simulink model "Test_thermal_rectifier_Werl"  (R2022a)
settings: Solver=VariableStepAuto  StartTime=0.0  StopTime=1000.0  RelTol=1e-3
libraries: nesl_utility x9
settings Model: Creator=Ravi  LastModifiedBy=Ravi

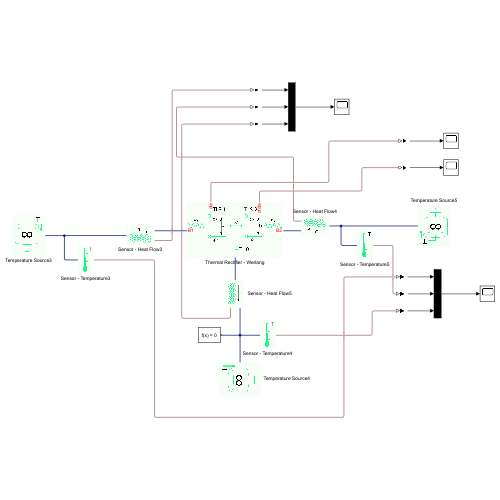
[thumbnail: Simulink's stored preview of the top-level diagram]
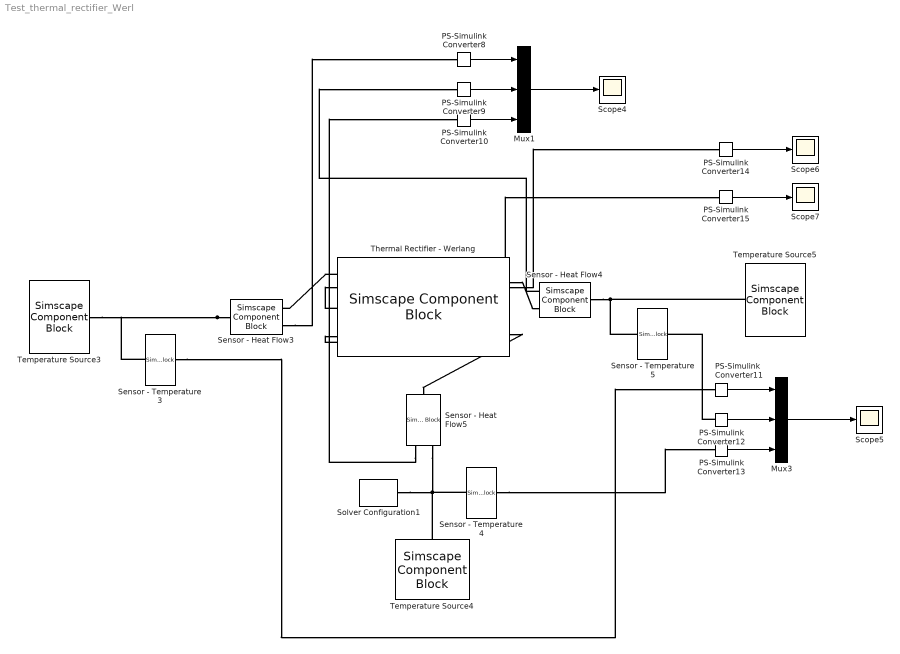
== system Test_thermal_rectifier_Werl ==
  Mux1 : Mux  Inputs=3
  Mux3 : Mux  Inputs=3
  PS-Simulink Converter{8..15} (8 alike) : nesl_utility/PS-Simulink Converter  PhysicalDomain=network_engine_domain  SubClassName=ps_output  LeftPortType=input  RightPortType=output  PseudoPeriodic=off  Frequencies=[]  VectorFormat=inherit  Unit=inherit  AffineConversion=off
      settings: SourceProductBaseCode=SS,PW,VE
  Scope{4..7} (4 alike) : Scope
  Sensor - Heat Flow3 : SimscapeComponentBlock  SourceFile=sensor_heat_flow  ComponentPath=sensor_heat_flow  ComponentVariants="[\"sensor_heat_flow\"]"  ComponentVariantNames="[\"sensor_heat_flow\"]"  ClassName=sensor_heat_flow  SchemaVersion=1  J_specify=off  J_priority=None  J=0  J_nominal_specify=off  J_nominal_unit=1  J_nominal_value=1
      settings: CopyFcn=simscape.engine.sli.internal.componentblockcallback(gcbh,'COPY')  PreCopyFcn=simscape.engine.sli.internal.componentblockcallback(gcbh,'PRECOPY')  PreDeleteFcn=simscape.engine.sli.internal.componentblockcallback(gcbh,'PREDELETE')  InternalSimscapePortConfiguration="{\"Bottom\":[],\"Left\":[{\"id\":\"inp\",\"label\":\"\",\"type\":\"quantum_thermal\"}],\"Right\":[{\"id\":\"out\",\"label\":\"\",\"type\":\"quantum_thermal\"},{\"id\":\"sense\",\"label\":\"\",\"type\":\"output\"}],\"Top\":[]}"
      mask Type: Heat flow rate sensor
  Sensor - Heat Flow4 : SimscapeComponentBlock  SourceFile=sensor_heat_flow  ComponentPath=sensor_heat_flow  ComponentVariants="[\"sensor_heat_flow\"]"  ComponentVariantNames="[\"sensor_heat_flow\"]"  ClassName=sensor_heat_flow  SchemaVersion=1  J_specify=off  J_priority=None  J=0  J_nominal_specify=off  J_nominal_unit=1  J_nominal_value=1
      settings: CopyFcn=simscape.engine.sli.internal.componentblockcallback(gcbh,'COPY')  PreCopyFcn=simscape.engine.sli.internal.componentblockcallback(gcbh,'PRECOPY')  PreDeleteFcn=simscape.engine.sli.internal.componentblockcallback(gcbh,'PREDELETE')  InternalSimscapePortConfiguration="{\"Bottom\":[],\"Left\":[{\"id\":\"inp\",\"label\":\"\",\"type\":\"quantum_thermal\"}],\"Right\":[{\"id\":\"out\",\"label\":\"\",\"type\":\"quantum_thermal\"},{\"id\":\"sense\",\"label\":\"\",\"type\":\"output\"}],\"Top\":[]}"
      mask Type: Heat flow rate sensor
  Sensor - Heat Flow5 : SimscapeComponentBlock  SourceFile=sensor_heat_flow  ComponentPath=sensor_heat_flow  ComponentVariants="[\"sensor_heat_flow\"]"  ComponentVariantNames="[\"sensor_heat_flow\"]"  ClassName=sensor_heat_flow  SchemaVersion=1  J_specify=off  J_priority=None  J=0  J_nominal_specify=off  J_nominal_unit=1  J_nominal_value=1
      settings: CopyFcn=simscape.engine.sli.internal.componentblockcallback(gcbh,'COPY')  PreCopyFcn=simscape.engine.sli.internal.componentblockcallback(gcbh,'PRECOPY')  PreDeleteFcn=simscape.engine.sli.internal.componentblockcallback(gcbh,'PREDELETE')  InternalSimscapePortConfiguration="{\"Bottom\":[],\"Left\":[{\"id\":\"inp\",\"label\":\"\",\"type\":\"quantum_thermal\"}],\"Right\":[{\"id\":\"out\",\"label\":\"\",\"type\":\"quantum_thermal\"},{\"id\":\"sense\",\"label\":\"\",\"type\":\"output\"}],\"Top\":[]}"
      mask Type: Heat flow rate sensor
  Sensor - Temperature3 : SimscapeComponentBlock  SourceFile=sensor_temperature  ComponentPath=sensor_temperature  ComponentVariants="[\"sensor_temperature\"]"  ComponentVariantNames="[\"sensor_temperature\"]"  ClassName=sensor_temperature  SchemaVersion=1  J_specify=off  J_priority=None  J=0  J_nominal_specify=off  J_nominal_unit=1  J_nominal_value=1
      settings: CopyFcn=simscape.engine.sli.internal.componentblockcallback(gcbh,'COPY')  PreCopyFcn=simscape.engine.sli.internal.componentblockcallback(gcbh,'PRECOPY')  PreDeleteFcn=simscape.engine.sli.internal.componentblockcallback(gcbh,'PREDELETE')  InternalSimscapePortConfiguration="{\"Bottom\":[],\"Left\":[{\"id\":\"inp\",\"label\":\"\",\"type\":\"quantum_thermal\"}],\"Right\":[{\"id\":\"sense\",\"label\":\"\",\"type\":\"output\"}],\"Top\":[]}"
      mask Type: Temperature sensor
  Sensor - Temperature4 : SimscapeComponentBlock  SourceFile=sensor_temperature  ComponentPath=sensor_temperature  ComponentVariants="[\"sensor_temperature\"]"  ComponentVariantNames="[\"sensor_temperature\"]"  ClassName=sensor_temperature  SchemaVersion=1  J_specify=off  J_priority=None  J=0  J_nominal_specify=off  J_nominal_unit=1  J_nominal_value=1
      settings: CopyFcn=simscape.engine.sli.internal.componentblockcallback(gcbh,'COPY')  PreCopyFcn=simscape.engine.sli.internal.componentblockcallback(gcbh,'PRECOPY')  PreDeleteFcn=simscape.engine.sli.internal.componentblockcallback(gcbh,'PREDELETE')  InternalSimscapePortConfiguration="{\"Bottom\":[],\"Left\":[{\"id\":\"inp\",\"label\":\"\",\"type\":\"quantum_thermal\"}],\"Right\":[{\"id\":\"sense\",\"label\":\"\",\"type\":\"output\"}],\"Top\":[]}"
      mask Type: Temperature sensor
  Sensor - Temperature5 : SimscapeComponentBlock  SourceFile=sensor_temperature  ComponentPath=sensor_temperature  ComponentVariants="[\"sensor_temperature\"]"  ComponentVariantNames="[\"sensor_temperature\"]"  ClassName=sensor_temperature  SchemaVersion=1  J_specify=off  J_priority=None  J=0  J_nominal_specify=off  J_nominal_unit=1  J_nominal_value=1
      settings: CopyFcn=simscape.engine.sli.internal.componentblockcallback(gcbh,'COPY')  PreCopyFcn=simscape.engine.sli.internal.componentblockcallback(gcbh,'PRECOPY')  PreDeleteFcn=simscape.engine.sli.internal.componentblockcallback(gcbh,'PREDELETE')  InternalSimscapePortConfiguration="{\"Bottom\":[],\"Left\":[{\"id\":\"inp\",\"label\":\"\",\"type\":\"quantum_thermal\"}],\"Right\":[{\"id\":\"sense\",\"label\":\"\",\"type\":\"output\"}],\"Top\":[]}"
      mask Type: Temperature sensor
  Solver Configuration1 : nesl_utility/Solver Configuration  PhysicalDomain=network_engine_domain  SubClassName=solver  LeftPortType=input  RightPortType=generic  Tones=[]  Harmonics=[]  SimulateNoise=off  Profile=off  UseLocalSampling=off  EnableSwitchedLinearOptims=on  FrequencyDomain=off  UseCCode=off  RelTol=0.001  AbsTol=0.001  MinStep=1e-09  ToWorkspace=off  RevertToSquareIcSolve=off  NumHomotopyIterations=100  PhasorMode=off  PhasorModeNumHarmonics=1  IndexReductionMethod=DerivativeReplacement  DoDC=off  ResidualTolerance=1e-09  UseLocalSolver=off  LocalSolverChoice=NE_BACKWARD_EULER_ADVANCER  LocalSolverSampleTime=0.001  DoFixedCost=off  MaxNonlinIter=3  MaxModeIter=2  ComputeImpulses=off  ImpulseIterations=2  LinearAlgebra=auto  LinearAlgebraNumThread=0  EquationFormulation=NE_TIME_EF  DelaysMemoryBudget=1024  AutomaticFiltering=on  FilteringTimeConstant=0.001  PartitionStorageMethod=AS_NEEDED  PartitionMemoryBudget=1024  PartitionMethod=ROBUST
      settings: SourceProductBaseCode=SS,PW,VE
  Temperature Source3 : SimscapeComponentBlock  SourceFile=source_temperature  ComponentPath=source_temperature  ComponentVariants="[\"source_temperature\"]"  ComponentVariantNames="[\"source_temperature\"]"  ClassName=source_temperature  SchemaVersion=1  temp=1  J_specify=off  J_priority=None  J=0  J_nominal_specify=off  J_nominal_unit=1  J_nominal_value=1
      settings: CopyFcn=simscape.engine.sli.internal.componentblockcallback(gcbh,'COPY')  PreCopyFcn=simscape.engine.sli.internal.componentblockcallback(gcbh,'PRECOPY')  PreDeleteFcn=simscape.engine.sli.internal.componentblockcallback(gcbh,'PREDELETE')  InternalSimscapePortConfiguration="{\"Bottom\":[],\"Left\":[],\"Right\":[{\"id\":\"out\",\"label\":\"\",\"type\":\"quantum_thermal\"}],\"Top\":[]}"
      mask Type: Temperature source
  Temperature Source4 : SimscapeComponentBlock  SourceFile=source_temperature  ComponentPath=source_temperature  ComponentVariants="[\"source_temperature\"]"  ComponentVariantNames="[\"source_temperature\"]"  ClassName=source_temperature  SchemaVersion=1  temp=0  J_specify=off  J_priority=None  J=0  J_nominal_specify=off  J_nominal_unit=1  J_nominal_value=1
      settings: CopyFcn=simscape.engine.sli.internal.componentblockcallback(gcbh,'COPY')  PreCopyFcn=simscape.engine.sli.internal.componentblockcallback(gcbh,'PRECOPY')  PreDeleteFcn=simscape.engine.sli.internal.componentblockcallback(gcbh,'PREDELETE')  InternalSimscapePortConfiguration="{\"Bottom\":[],\"Left\":[],\"Right\":[{\"id\":\"out\",\"label\":\"\",\"type\":\"quantum_thermal\"}],\"Top\":[]}"
      mask Type: Temperature source
  Temperature Source5 : SimscapeComponentBlock  SourceFile=source_temperature  ComponentPath=source_temperature  ComponentVariants="[\"source_temperature\"]"  ComponentVariantNames="[\"source_temperature\"]"  ClassName=source_temperature  SchemaVersion=1  temp=0.3  J_specify=off  J_priority=None  J=0  J_nominal_specify=off  J_nominal_unit=1  J_nominal_value=1
      settings: CopyFcn=simscape.engine.sli.internal.componentblockcallback(gcbh,'COPY')  PreCopyFcn=simscape.engine.sli.internal.componentblockcallback(gcbh,'PRECOPY')  PreDeleteFcn=simscape.engine.sli.internal.componentblockcallback(gcbh,'PREDELETE')  InternalSimscapePortConfiguration="{\"Bottom\":[],\"Left\":[],\"Right\":[{\"id\":\"out\",\"label\":\"\",\"type\":\"quantum_thermal\"}],\"Top\":[]}"
      mask Type: Temperature source
  Thermal Rectifier - Werlang : SimscapeComponentBlock  SourceFile=thermal_rectifier_Werl  ComponentPath=thermal_rectifier_Werl  ComponentVariants="[\"thermal_rectifier_Werl\"]"  ComponentVariantNames="[\"thermal_rectifier_Werl\"]"  ClassName=thermal_rectifier_Werl  SchemaVersion=1  k1=0.01  k2=0.01  w=1  d=0.5  p11_specify=off  p11_priority=High  p11=0  p11_nominal_specify=off  p11_nominal_unit=1  p11_nominal_value=1  p22_specify=off  p22_priority=High  p22=0  p22_nominal_specify=off  p22_nominal_unit=1  p22_nominal_value=1  p33_specify=off  p33_priority=High  p33=0  p33_nominal_specify=off  p33_nominal_unit=1  p33_nominal_value=1  p44_specify=off  p44_priority=High  p44=1  p44_nominal_specify=off  p44_nominal_unit=1  p44_nominal_value=1  T1_specify=off  T1_priority=Low  T1=0.2  T1_nominal_specify=off  T1_nominal_unit=1  T1_nominal_value=1  T2_specify=off  T2_priority=Low  T2=0.2  T2_nominal_specify=off  T2_nominal_unit=1  T2_nominal_value=1  J1_specify=off  J1_priority=Low  J1=0  J1_nominal_specify=off  J1_nominal_unit=1  J1_nominal_value=1  J2_specify=off  J2_priority=Low  J2=0  J2_nominal_specify=off  J2_nominal_unit=1  J2_nominal_value=1
      settings: CopyFcn=simscape.engine.sli.internal.componentblockcallback(gcbh,'COPY')  PreCopyFcn=simscape.engine.sli.internal.componentblockcallback(gcbh,'PRECOPY')  PreDeleteFcn=simscape.engine.sli.internal.componentblockcallback(gcbh,'PREDELETE')  InternalSimscapePortConfiguration="{\"Bottom\":[{\"id\":\"gnd\",\"label\":\"\",\"type\":\"quantum_thermal\"}],\"Left\":[{\"id\":\"b1\",\"label\":\"B1\",\"type\":\"quantum_thermal\"}],\"Right\":[{\"id\":\"b2\",\"label\":\"B2\",\"type\":\"quantum_thermal\"}],\"Top\":[{\"id\":\"diag\",\"label\":\"dia\",\"type\":\"output\"},{\"id\":\"ofdiag\",\"label\":\"ofdia\",\"type\":\"output\"}]}"
      mask Type: Thermal rectifier
  wires:
  PS-Simulink Converter15/1 -> Scope7/1
  PS-Simulink Converter14/1 -> Scope6/1
  Mux3/1 -> Scope5/1
  Mux1/1 -> Scope4/1
  PS-Simulink Converter8/1 -> Mux1/1
  PS-Simulink Converter9/1 -> Mux1/2
  PS-Simulink Converter10/1 -> Mux1/3
  PS-Simulink Converter11/1 -> Mux3/1
  PS-Simulink Converter12/1 -> Mux3/2
  PS-Simulink Converter13/1 -> Mux3/3
  connections:
  Sensor - Heat Flow3/LConn1 -- Temperature Source3/RConn1 -- Sensor - Temperature3/LConn1
  Sensor - Heat Flow4/LConn1 -- Temperature Source5/RConn1 -- Sensor - Temperature5/LConn1
  Sensor - Heat Flow5/RConn1 -- Temperature Source4/RConn1 -- Solver Configuration1/RConn1 -- Sensor - Temperature4/LConn1
  Thermal Rectifier - Werlang/LConn3 -- PS-Simulink Converter15/LConn1
  Thermal Rectifier - Werlang/LConn2 -- PS-Simulink Converter14/LConn1
  Sensor - Heat Flow5/RConn2 -- PS-Simulink Converter10/LConn1
  Sensor - Heat Flow4/RConn2 -- PS-Simulink Converter9/LConn1
  Sensor - Heat Flow3/RConn2 -- PS-Simulink Converter8/LConn1
  Sensor - Temperature4/RConn1 -- PS-Simulink Converter13/LConn1
  Sensor - Temperature3/RConn1 -- PS-Simulink Converter11/LConn1
  Thermal Rectifier - Werlang/RConn1 -- Sensor - Heat Flow4/RConn1
  Thermal Rectifier - Werlang/LConn1 -- Sensor - Heat Flow3/RConn1
  PS-Simulink Converter12/LConn1 -- Sensor - Temperature5/RConn1
  Thermal Rectifier - Werlang/RConn2 -- Sensor - Heat Flow5/LConn1
